simulink model "yeon_Ultra_to_Dcmotor"  (R2022b)
settings: Solver=VariableStepAuto  StartTime=0.0  StopTime=10.0  RelTol=1e-3
libraries: arduinolib x1, arduinosensorlib x1
settings Model: Creator=user  LastModifiedBy=user

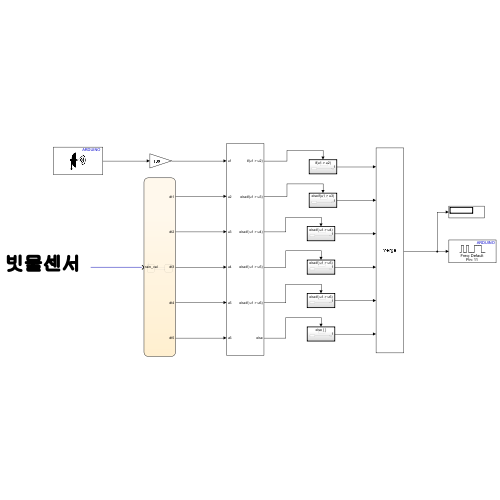
[thumbnail: Simulink's stored preview of the top-level diagram]
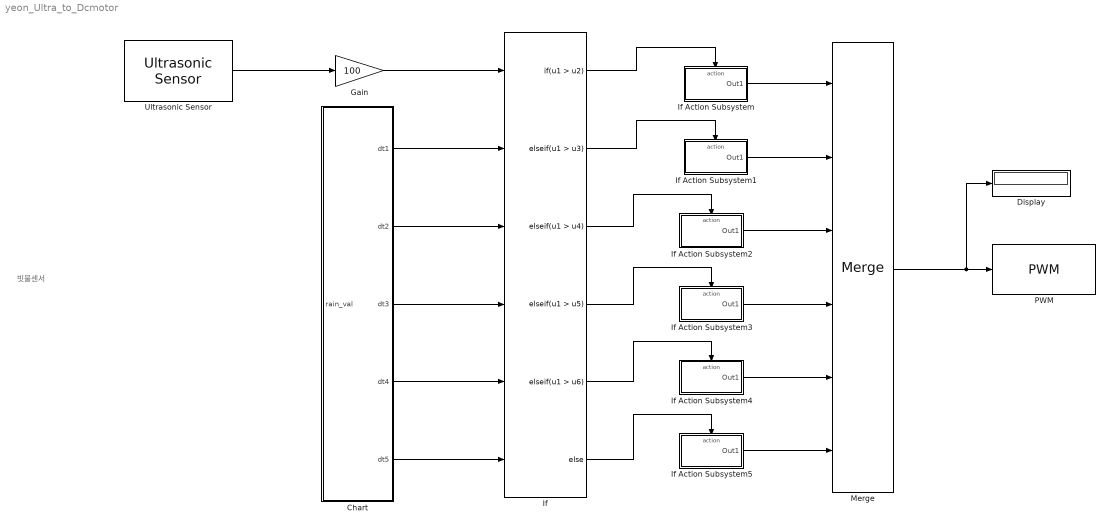
== system yeon_Ultra_to_Dcmotor ==
  note: 빗물센서
  Chart : Stateflow chart  TreatAsAtomicUnit=on
  Display : Display
  Gain : Gain  Gain=100
  If : If  NumInputs=6  IfExpression=u1 > u2  ElseIfExpressions=u1 > u3, u1 > u4, u1 > u5, u1 > u6
  If Action Subsystem : Subsystem  TreatAsAtomicUnit=on
  If Action Subsystem1 : Subsystem  TreatAsAtomicUnit=on
  If Action Subsystem2 : Subsystem  TreatAsAtomicUnit=on
  If Action Subsystem3 : Subsystem  TreatAsAtomicUnit=on
  If Action Subsystem4 : Subsystem  TreatAsAtomicUnit=on
  If Action Subsystem5 : Subsystem  TreatAsAtomicUnit=on
  Merge : Merge  Inputs=6
  PWM : arduinolib/PWM  pinNumber=11  frequencyType=Default  desiredFrequency=490.2  achievableFrequency=490.2
  Ultrasonic Sensor : arduinosensorlib/Ultrasonic Sensor  NumSignalPins=1  TrigPin=4  EchoPin=5  SignalPin=3  SampleTime_=0.1  blockPlatform=ARDUINO
  wires:
  Ultrasonic Sensor/1 -> Gain/1
  Chart/1(dt1) -> If/2
  Chart/2(dt2) -> If/3
  Chart/3(dt3) -> If/4
  Chart/5(dt5) -> If/6
  Chart/4(dt4) -> If/5
  If Action Subsystem/1(Out1) -> Merge/1
  Gain/1 -> If/1
  If/2 -> If Action Subsystem1/Action
  If/3 -> If Action Subsystem2/Action
  If/4 -> If Action Subsystem3/Action
  If/5 -> If Action Subsystem4/Action
  If/6 -> If Action Subsystem5/Action
  If/1 -> If Action Subsystem/Action
  If Action Subsystem1/1(Out1) -> Merge/2
  If Action Subsystem2/1(Out1) -> Merge/3
  If Action Subsystem3/1(Out1) -> Merge/4
  If Action Subsystem4/1(Out1) -> Merge/5
  If Action Subsystem5/1(Out1) -> Merge/6
  Merge/1 -> Display/1, PWM/1

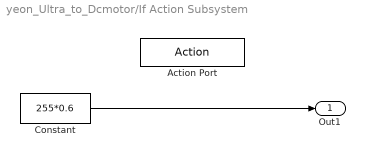
== system yeon_Ultra_to_Dcmotor/If Action Subsystem ==
  Action Port : ActionPort  ActionPortLabel=if(u1 > u2)
  Constant : Constant  Value=255*0.6
  Out1 : Outport
  wires:
  Constant/1 -> Out1/1

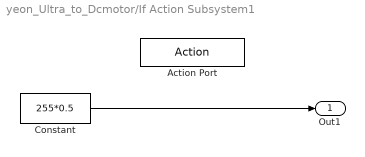
== system yeon_Ultra_to_Dcmotor/If Action Subsystem1 ==
  Action Port : ActionPort  ActionPortLabel=elseif(u1 > u3)
  Constant : Constant  Value=255*0.5
  Out1 : Outport
  wires:
  Constant/1 -> Out1/1

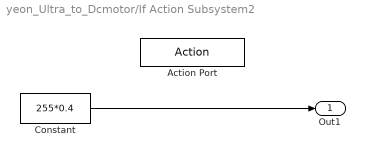
== system yeon_Ultra_to_Dcmotor/If Action Subsystem2 ==
  Action Port : ActionPort  ActionPortLabel=elseif( u1 > u4)
  Constant : Constant  Value=255*0.4
  Out1 : Outport
  wires:
  Constant/1 -> Out1/1

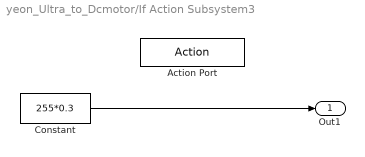
== system yeon_Ultra_to_Dcmotor/If Action Subsystem3 ==
  Action Port : ActionPort  ActionPortLabel=elseif( u1 > u5)
  Constant : Constant  Value=255*0.3
  Out1 : Outport
  wires:
  Constant/1 -> Out1/1

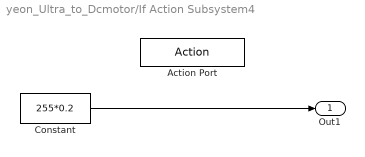
== system yeon_Ultra_to_Dcmotor/If Action Subsystem4 ==
  Action Port : ActionPort  ActionPortLabel=elseif( u1 > u6)
  Constant : Constant  Value=255*0.2
  Out1 : Outport
  wires:
  Constant/1 -> Out1/1

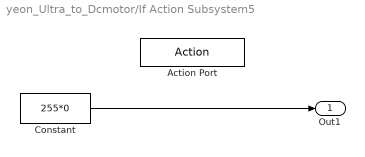
== system yeon_Ultra_to_Dcmotor/If Action Subsystem5 ==
  Action Port : ActionPort  ActionPortLabel=else
  Constant : Constant  Value=255*0
  Out1 : Outport
  wires:
  Constant/1 -> Out1/1

== stateflow chart yeon_Ultra_to_Dcmotor/Chart ==
  state Non_rain
    dt1 = 50
    dt2 = 40
    dt3 = 30
    dt4 = 20
    dt5 = 10
  state Rain
    dt1=55
    dt2=45
    dt3=35
    dt4=25
    dt5=15
  (default) -> Non_rain
  Rain -> Non_rain : [rain_val > 800]
  Non_rain -> Rain : [rain_val <= 800]
  data: dt1 output; dt2 output; dt3 output; dt4 output; dt5 output; rain_val input
